simulink model "hydraulic_ex3"  (R2015b)
settings: Solver=VariableStepAuto  StartTime=0.0  StopTime=simtime  RelTol=1e-3
values from neighbouring files (symbols this model uses):
  A = s+b    [Task3Sensitivity.m]    (also in Velocity_ctrl_HYDRAULIC.m = [-df/m Am/m -Am/m; t3s.m = tf(Go.den{1}, [1]))
  A1 = Am    (= 0.00180641577581)    [Velocity_ctrl_HYDRAULIC.m]
  A2 = Am    (= 0.00180641577581)    [Velocity_ctrl_HYDRAULIC.m]
  B = a    (= 25.15)    [Task3Sensitivity.m]    (also in Velocity_ctrl_HYDRAULIC.m = [ 0; t3s.m = tf(Go.num{1}, [1]))
  C = [1 0 0]    [Velocity_ctrl_HYDRAULIC.m]
  Cf = Volume0/B    (= 6.87223392973e-13)    [Velocity_ctrl_HYDRAULIC.m]
  D = [0]    [Velocity_ctrl_HYDRAULIC.m]
  df = uf    (= 200)    [Velocity_ctrl_HYDRAULIC.m]
  Fe = 5000    [Velocity_ctrl_HYDRAULIC.m]
  G = minreal(tf(NUM,DEN))    [Velocity_ctrl_HYDRAULIC.m]
  m = 200    [Velocity_ctrl_HYDRAULIC.m]
  p10 = double(solution.p1)    [Velocity_ctrl_HYDRAULIC.m]
  p20 = double(solution.p2)    [Velocity_ctrl_HYDRAULIC.m]
  Ps = 20e6    (= 20000000)    [Velocity_ctrl_HYDRAULIC.m]
  R = s    [Task3Sensitivity.m]    (also in Velocity_ctrl_HYDRAULIC.m = s*(s+r0); t3s.m = tf(R_vector, [1]))
  Rv = 1e-4    (= 0.0001)    [Velocity_ctrl_HYDRAULIC.m]
  S = c*s+d    [Task3Sensitivity.m]    (also in Velocity_ctrl_HYDRAULIC.m = s^2*s2+s*s1+s0; t3s.m = tf(S_vector, [1]))
  T = t0*Ao    [Task3Sensitivity.m]    (also in Velocity_ctrl_HYDRAULIC.m = t0*(2*Zeta2*omega2*s+omega2^2+s^2); t3s.m = tf(T_vector, [1]))
  Tforce = 0.03    [Velocity_ctrl_HYDRAULIC.m]
  xv = 0.003    [Velocity_ctrl_HYDRAULIC.m]
settings Model: Creator=gabri  LastModifiedBy=Gabriel
settings SolverCC: ZeroCrossAlgorithm=Adaptive

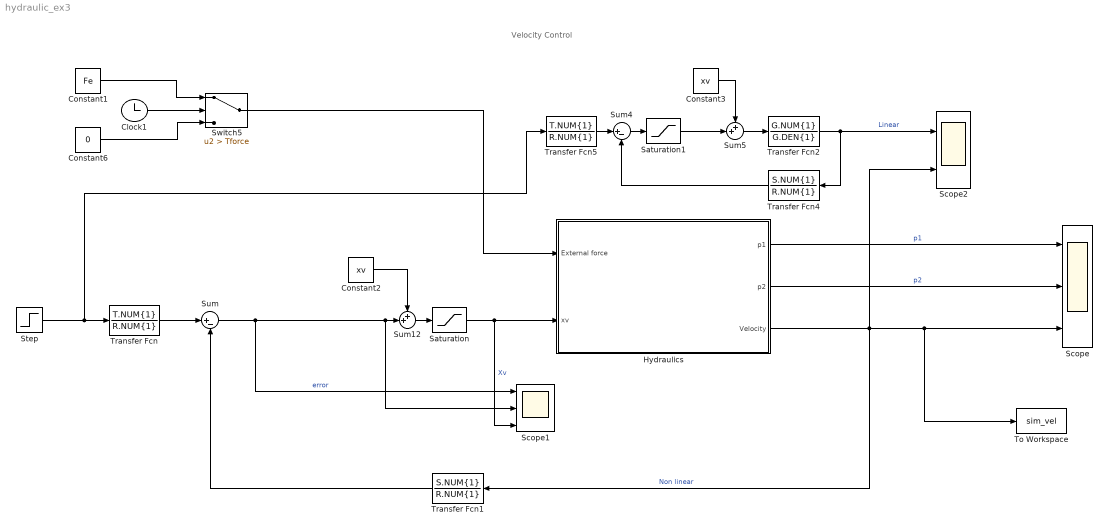
== system hydraulic_ex3 ==
  note: Velocity Control
  Clock1 : Clock
  Constant1 : Constant  Value=Fe
  Constant2 : Constant  Value=xv
  Constant3 : Constant  Value=xv
  Constant6 : Constant  Value=0
  "Hydraulics " : Subsystem
  Saturation : Saturate  UpperLimit=0.01  LowerLimit=-0.01
  Saturation1 : Saturate  UpperLimit=0.01  LowerLimit=-0.01
  Scope : Scope  NumInputPorts=3
  Scope1 : Scope  NumInputPorts=3
  Scope2 : Scope  NumInputPorts=2
  Step : Step  Time=0  After=0.5  SampleTime=0
  Sum : Sum  Inputs=|+-
  Sum12 : Sum  Inputs=++|
  Sum4 : Sum  Inputs=|+-
  Sum5 : Sum  Inputs=++|
  Switch5 : Switch  Criteria=u2 > Threshold  Threshold=Tforce
  To Workspace : ToWorkspace  VariableName=sim_vel  SaveFormat=Timeseries  SampleTime=-1
  Transfer Fcn : TransferFcn  Numerator=T.NUM{1}  Denominator=R.NUM{1}
  Transfer Fcn1 : TransferFcn  Numerator=S.NUM{1}  Denominator=R.NUM{1}
  Transfer Fcn2 : TransferFcn  Numerator=G.NUM{1}  Denominator=G.DEN{1}
  Transfer Fcn4 : TransferFcn  Numerator=S.NUM{1}  Denominator=R.NUM{1}
  Transfer Fcn5 : TransferFcn  Numerator=T.NUM{1}  Denominator=R.NUM{1}
  wires:
  Clock1/1 -> Switch5/2
  Constant1/1 -> Switch5/1
  Constant6/1 -> Switch5/3
  "Hydraulics "/1(p1) -> Scope/1  "p1"
  "Hydraulics "/2(p2) -> Scope/2  "p2"
  "Hydraulics "/3(Velocity) -> Transfer Fcn1/1, To Workspace/1, Scope/3, Scope2/2  "Non linear"
  Sum/1 -> Scope1/2, Sum12/2, Scope1/1  "error"
  Saturation/1 -> "Hydraulics "/2(xv), Scope1/3  "Xv"
  Switch5/1 -> "Hydraulics "/1(External force)
  Step/1 -> Transfer Fcn5/1, Transfer Fcn/1
  Constant2/1 -> Sum12/1
  Transfer Fcn/1 -> Sum/1
  Transfer Fcn1/1 -> Sum/2
  Transfer Fcn2/1 -> Transfer Fcn4/1, Scope2/1  "Linear"
  Transfer Fcn4/1 -> Sum4/2
  Sum4/1 -> Saturation1/1
  Transfer Fcn5/1 -> Sum4/1
  Saturation1/1 -> Sum5/2
  Sum5/1 -> Transfer Fcn2/1
  Constant3/1 -> Sum5/1
  Sum12/1 -> Saturation/1

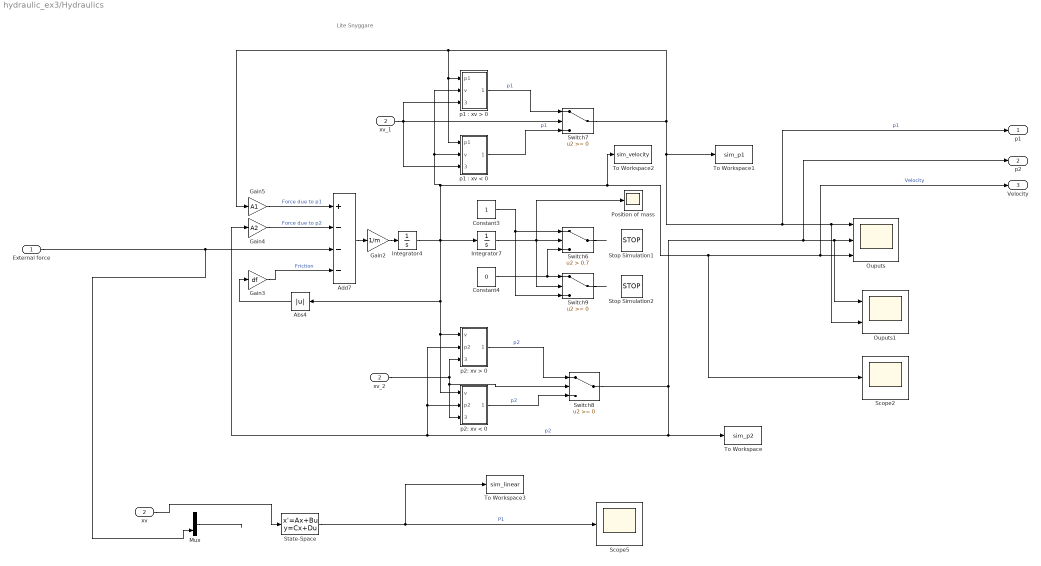
== system hydraulic_ex3/Hydraulics  ==
  note: Lite Snyggare
  External force : Inport
  xv : Inport  Port=2
  Abs4 : Abs
  Add7 : Sum  Inputs=+---
  Constant3 : Constant
  Constant4 : Constant  Value=0
  Gain2 : Gain  Gain=1/m
  Gain3 : Gain  Gain=df
  Gain4 : Gain  Gain=A2
  Gain5 : Gain  Gain=A1
  Integrator4 : Integrator
  Integrator7 : Integrator
  Mux : Mux  Inputs=2
  Ouputs : Scope  NumInputPorts=3
  Ouputs1 : Scope  NumInputPorts=2
  Position of mass : Scope
  Scope2 : Scope
  Scope5 : Scope
  State-Space : StateSpace  A=A  B=B  C=C  D=D  X0=0
  Stop Simulation1 : Stop
  Stop Simulation2 : Stop
  Switch6 : Switch  Criteria=u2 > Threshold  Threshold=0.7
  Switch7 : Switch
  Switch8 : Switch
  Switch9 : Switch
  To Workspace : ToWorkspace  VariableName=sim_p2  SaveFormat=Timeseries  SampleTime=-1
  To Workspace1 : ToWorkspace  VariableName=sim_p1  SaveFormat=Timeseries  SampleTime=-1
  To Workspace2 : ToWorkspace  VariableName=sim_velocity  SaveFormat=Timeseries  SampleTime=-1
  To Workspace3 : ToWorkspace  VariableName=sim_linear  SaveFormat=Timeseries  SampleTime=-1
  "p1 : xv < 0" : Subsystem
  "p1 : xv > 0" : Subsystem
  p2: xv < 0 : Subsystem
  "p2: xv > 0 " : Subsystem
  xv_1 : InportShadow  Port=2
  xv_2 : InportShadow  Port=2
  p1 : Outport
  p2 : Outport  Port=2
  Velocity : Outport  Port=3
  wires:
  Switch7/1 -> p1/1, Ouputs1/2, Ouputs/1, To Workspace1/1, "p1 : xv < 0"/1(p1), "p1 : xv > 0"/1("p1 "), Gain5/1  "p1"
  Gain2/1 -> Integrator4/1
  xv_2/1 -> p2: xv < 0/3(xv_1), Switch8/2, "p2: xv > 0 "/3(xv_1)
  Mux/1 -> ?
  Constant3/1 -> Switch9/3, Switch6/1
  "p1 : xv > 0"/1(Out1) -> Switch7/1  "p1"
  Add7/1 -> Gain2/1
  Integrator7/1 -> Position of mass/1, Switch6/2, Switch9/2
  xv/1 -> State-Space/1
  Switch8/1 -> p2/1, Ouputs1/1, Ouputs/2, To Workspace/1, p2: xv < 0/2(p2), "p2: xv > 0 "/2(p2), Gain4/1  "p2"
  External force/1 -> Mux/2, Add7/3
  "p2: xv > 0 "/1(Out1) -> Switch8/1  "p2"
  xv_1/1 -> "p1 : xv < 0"/3(xv_1), "p1 : xv > 0"/3(xv_1), Switch7/2
  Integrator4/1 -> Integrator7/1, "p1 : xv < 0"/2(v), "p1 : xv > 0"/2(v), Scope2/1, Velocity/1, Ouputs/3, To Workspace2/1, Abs4/1, p2: xv < 0/1(v), "p2: xv > 0 "/1(v)  "Velocity"
  Abs4/1 -> Gain3/1
  Gain3/1 -> Add7/4  "Friction"
  Gain5/1 -> Add7/1  "Force due to p1"
  p2: xv < 0/1(Out1) -> Switch8/3  "p2"
  Constant4/1 -> Switch6/3, Switch9/1
  Gain4/1 -> Add7/2  "Force due to p2"
  State-Space/1 -> Scope5/1, To Workspace3/1  "P1"
  Switch6/1 -> ?
  Switch9/1 -> ?
  "p1 : xv < 0"/1(Out1) -> Switch7/3  "p1"

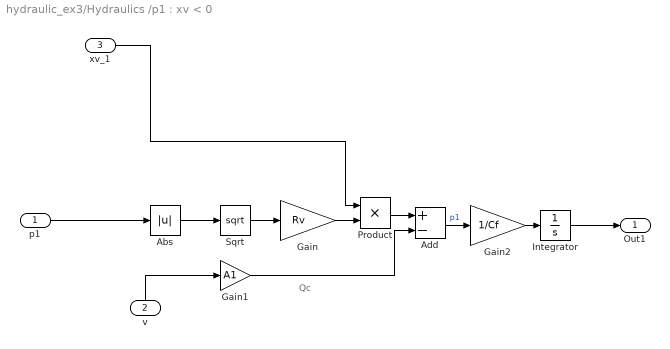
== system hydraulic_ex3/Hydraulics /p1 : xv < 0 ==
  note: Qc
  p1 : Inport
  v : Inport  Port=2
  xv_1 : Inport  Port=3
  Abs : Abs
  Add : Sum  Inputs=+-
  Gain : Gain  Gain=Rv
  Gain1 : Gain  Gain=A1
  Gain2 : Gain  Gain=1/Cf
  Integrator : Integrator
  Product : Product
  Sqrt : Sqrt  SaturateOnIntegerOverflow=on
  Out1 : Outport
  wires:
  v/1 -> Gain1/1
  Gain1/1 -> Add/2
  Abs/1 -> Sqrt/1
  p1/1 -> Abs/1
  Add/1 -> Gain2/1  "p1"
  Gain2/1 -> Integrator/1
  Integrator/1 -> Out1/1
  Sqrt/1 -> Gain/1
  Gain/1 -> Product/2
  xv_1/1 -> Product/1
  Product/1 -> Add/1

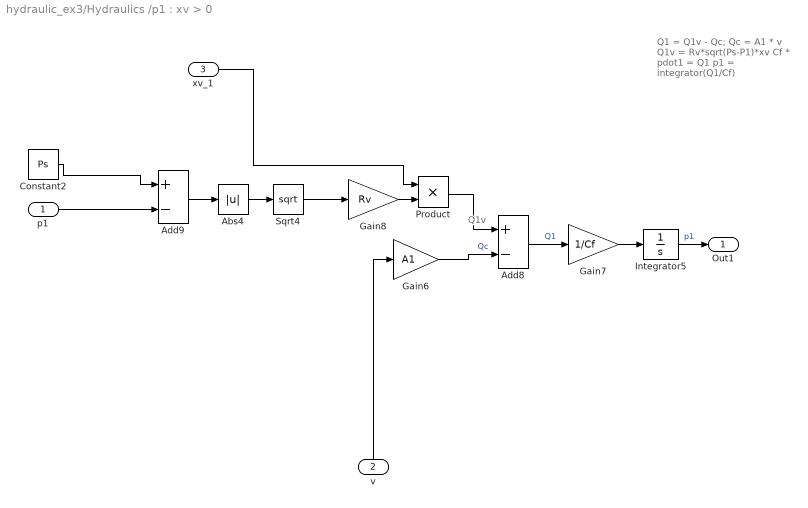
== system hydraulic_ex3/Hydraulics /p1 : xv > 0 ==
  note: Q1v
  note: Q1 = Q1v - Qc;
      | Qc = A1 * v
      | Q1v = Rv*sqrt(Ps-P1)*xv
      | Cf * pdot1 = Q1
      | p1 = integrator(Q1/Cf)
  "p1 " : Inport
  v : Inport  Port=2
  xv_1 : Inport  Port=3
  Abs4 : Abs
  Add8 : Sum  Inputs=+-
  Add9 : Sum  Inputs=+-
  Constant2 : Constant  Value=Ps
  Gain6 : Gain  Gain=A1
  Gain7 : Gain  Gain=1/Cf
  Gain8 : Gain  Gain=Rv
  Integrator5 : Integrator  InitialCondition=p10
  Product : Product
  Sqrt4 : Sqrt  SaturateOnIntegerOverflow=on
  Out1 : Outport
  wires:
  Add9/1 -> Abs4/1
  Constant2/1 -> Add9/1
  Abs4/1 -> Sqrt4/1
  Gain7/1 -> Integrator5/1
  Gain6/1 -> Add8/2  "Qc"
  Integrator5/1 -> Out1/1  "p1"
  Add8/1 -> Gain7/1  "Q1"
  Sqrt4/1 -> Gain8/1
  Gain8/1 -> Product/2
  v/1 -> Gain6/1
  "p1 "/1 -> Add9/2
  xv_1/1 -> Product/1
  Product/1 -> Add8/1

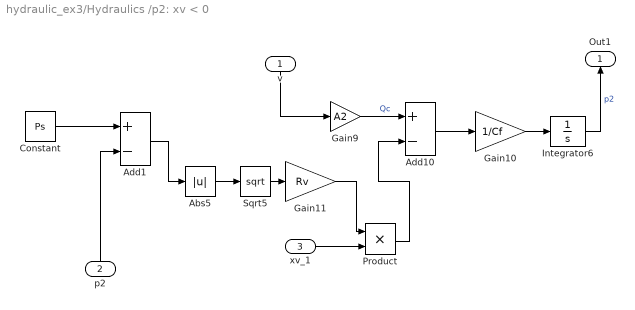
== system hydraulic_ex3/Hydraulics /p2: xv < 0 ==
  v : Inport
  p2 : Inport  Port=2
  xv_1 : Inport  Port=3
  Abs5 : Abs
  Add1 : Sum  Inputs=+-
  Add10 : Sum  Inputs=+-
  Constant : Constant  Value=Ps
  Gain10 : Gain  Gain=1/Cf
  Gain11 : Gain  Gain=Rv
  Gain9 : Gain  Gain=A2
  Integrator6 : Integrator
  Product : Product
  Sqrt5 : Sqrt  SaturateOnIntegerOverflow=on
  Out1 : Outport
  wires:
  Abs5/1 -> Sqrt5/1
  Gain9/1 -> Add10/1  "Qc"
  Sqrt5/1 -> Gain11/1
  Gain10/1 -> Integrator6/1
  Add10/1 -> Gain10/1
  Integrator6/1 -> Out1/1  "p2"
  v/1 -> Gain9/1
  p2/1 -> Add1/2
  Add1/1 -> Abs5/1
  Constant/1 -> Add1/1
  Product/1 -> Add10/2
  xv_1/1 -> Product/2
  Gain11/1 -> Product/1

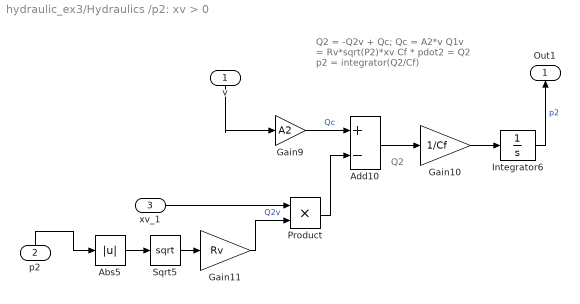
== system hydraulic_ex3/Hydraulics /p2: xv > 0  ==
  note: Q2
  note: Q2 = -Q2v + Qc;
      | Qc = A2*v
      | Q1v = Rv*sqrt(P2)*xv
      | Cf * pdot2 = Q2
      | p2 = integrator(Q2/Cf)
  v : Inport
  p2 : Inport  Port=2
  xv_1 : Inport  Port=3
  Abs5 : Abs
  Add10 : Sum  Inputs=+-
  Gain10 : Gain  Gain=1/Cf
  Gain11 : Gain  Gain=Rv
  Gain9 : Gain  Gain=A2
  Integrator6 : Integrator  InitialCondition=p20
  Product : Product
  Sqrt5 : Sqrt  SaturateOnIntegerOverflow=on
  Out1 : Outport
  wires:
  p2/1 -> Abs5/1
  v/1 -> Gain9/1
  Integrator6/1 -> Out1/1  "p2"
  Add10/1 -> Gain10/1
  Gain10/1 -> Integrator6/1
  Sqrt5/1 -> Gain11/1
  Gain11/1 -> Product/2  "Q2v"
  Gain9/1 -> Add10/1  "Qc"
  Abs5/1 -> Sqrt5/1
  xv_1/1 -> Product/1
  Product/1 -> Add10/2
